simulink model "Tavola3_tris_FL"  (R2018b)
settings: Solver=VariableStepAuto  StartTime=0.0  StopTime=50  RelTol=1e-3
settings Model: Creator=Utente  LastModifiedBy=giga4

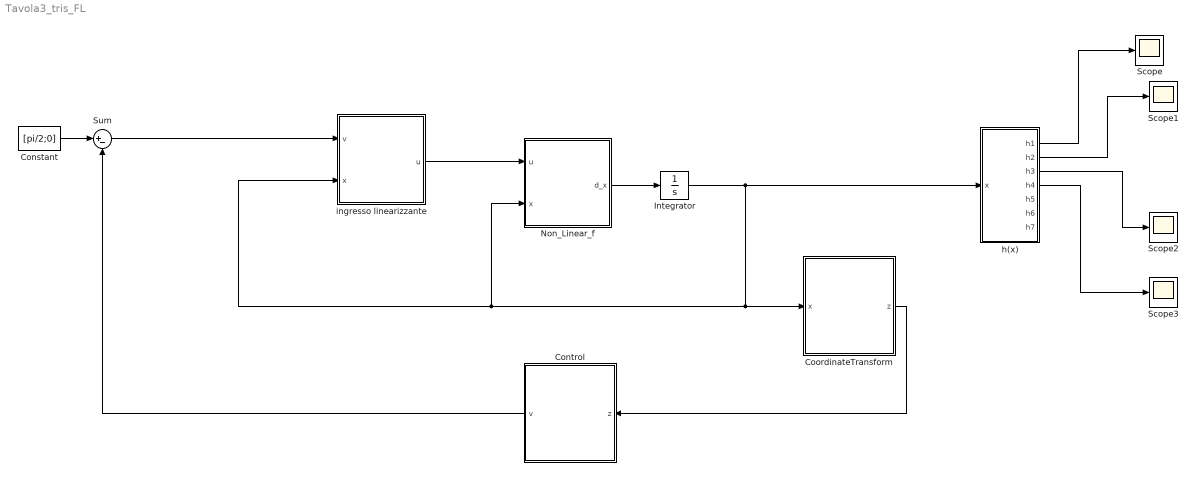
== system Tavola3_tris_FL ==
  Constant : Constant  Value=[pi/2;0]
  Control : MATLAB Function  TreatAsAtomicUnit=on
  CoordinateTransform : MATLAB Function  TreatAsAtomicUnit=on
  Integrator : Integrator  InitialCondition=[0,0,0,0.17,5,0,0]
  "Non_Linear_f " : MATLAB Function  TreatAsAtomicUnit=on
  Scope{,1..3} (4 alike) : Scope
  Sum : Sum  Inputs=|+-
  h(x) : MATLAB Function  TreatAsAtomicUnit=on
  ingresso linearizzante : MATLAB Function  TreatAsAtomicUnit=on
  wires:
  "Non_Linear_f "/1(d_x) -> Integrator/1
  Integrator/1 -> CoordinateTransform/1(x), "Non_Linear_f "/2(x), ingresso linearizzante/2(x), h(x)/1(x)
  h(x)/1(h1) -> Scope/1
  h(x)/2(h2) -> Scope1/1
  ingresso linearizzante/1(u) -> "Non_Linear_f "/1(u)
  Constant/1 -> Sum/1
  Sum/1 -> ingresso linearizzante/1(v)
  h(x)/3(h3) -> Scope2/1
  h(x)/4(h4) -> Scope3/1
  CoordinateTransform/1(z) -> Control/1(z)
  Control/1(v) -> Sum/2

== matlab function Tavola3_tris_FL/h(x) ==
  data: x input; h1 output; h2 output; h3 output; h4 output; h5 output; h6 output; h7 output
function [h1,h2,h3,h4,h5,h6,h7] = h(x)

x1 = x(1);
x2 = x(2);
x3 = x(3);
x4 = x(4);
x5 = x(5);
x6 = x(6);
x7 = x(7);


h1 = x1;
h2 = x2;
h3 = x3;
h4 = x4;
h5 = x5;
h6 = x6;
h7 = x7;

== matlab function Tavola3_tris_FL/Non_Linear_f  ==
  data: u input; d_x output; x input
function d_x = statespacef(u,x)

x1 = x(1);
x2 = x(2);
x3 = x(3);
x4 = x(4);
x5 = x(5);
x6 = x(6);
x7 = x(7);


f =                                                                                                                               [x6*cos(x3);
                                                                                                                                  x6*sin(x3);
                                                                                                                                          x7;
                                                                                                                                          x5;
 (2.39*sin(2.0*x4)*x5^2)/(4.79*cos(x4)^2 - 12.5) - (173.0*sin(x4))/(4.79*cos(x4)^2 - 12.5) - (3.28*x7^2*sin(2.0*x4))/(4.79*cos(x4)^2 - 12.5);
       (1.99*sin(3.0*x4) - 6.77*sin(x4))*x7^2 + (23.5*sin(2.0*x4))/(4.79*cos(x4)^2 - 12.5) - (2.19*x5^2*sin(2.0*x4))/(4.79*cos(x4)^2 - 12.5);
                                       (0.547*x6*x7*sin(x4))/(0.228*cos(x4)^2 - 0.315) + (0.228*x5*x7*sin(2.0*x4))/(0.228*cos(x4)^2 - 0.315)];
                                   
g1 =                        [0;
                             0;
                             0;
                             0;
      (35*cos(x3))/16 + 249/80;
 - (35*cos(x4))/64 - 1603/1600;
                             0];
g2 = [0;0;0;0;0;0;1];

d_x = f + [g1,g2]*u;

== matlab function Tavola3_tris_FL/ingresso linearizzante ==
  data: v input; u output; x input
function u = inputLinearizzante(v,x)

x1 = x(1);
x2 = x(2);
x3 = x(3);
x4 = x(4);
x5 = x(5);
x6 = x(6);
x7 = x(7);

inv_E =  [ 0, 80/(175*cos(x3) + 249);
           1,                      0];
       
Gamma =                               [(0.547*x6*x7*sin(x4))/(0.228*cos(x4)^2 - 0.315) + (0.228*x5*x7*sin(2.0*x4))/(0.228*cos(x4)^2 - 0.315);
 (2.39*sin(2.0*x4)*x5^2)/(4.79*cos(x4)^2 - 12.5) - (173.0*sin(x4))/(4.79*cos(x4)^2 - 12.5) - (3.28*x7^2*sin(2.0*x4))/(4.79*cos(x4)^2 - 12.5)];

u = -inv_E*Gamma+inv_E*v;

== matlab function Tavola3_tris_FL/CoordinateTransform ==
  data: z output; x input
function z = transformCoordinate(x)

x1 = x(1);
x2 = x(2);
x3 = x(3);
x4 = x(4);
x5 = x(5);
x6 = x(6);
x7 = x(7);

z =  [                                                         x3;
                                                               x7;
                                                               x4;
                                                               x5;
                                                               x1;
                                                               x2;
 x6*((35*cos(x3))/16 + 249/80) + x5*((35*cos(x4))/64 + 1603/160);];

== matlab function Tavola3_tris_FL/Control ==
  data: v output; z input
function v = control(z)

z1 = z(1);
z2 = z(2);
z3 = z(3);
z4 = z(4);
z5 = z(5);
z6 = z(6);
z7 = z(7);

k11 = 1;
k12 = 1;
k21 = 1;
k22 = 1;

v1 = k11*z1+k12*z2;
v2 = k21*z3+k22*z4;

v = [v1;v2];
